simulink model "Final_V620140905h5b_fuben1"  (Simulink 7.9)
settings: Solver=FixedStepDiscrete  StartTime=0.0  StopTime=1  FixedStep=Auto  RelTol=1e-3
undefined symbols (not defined in the file or in its folder): Down, Up
libraries: tiiqmathlib x157, idelinklib_common x83, c2833xlib x37, simulink x12, c28xdmclib x12, c280xlib x7, simulink_extras x4, commutil2 x2, idelinklib_tgtpref x1, idelinklib_ticcs x1
(part 3 of 7)

== system Final_V620140905h5b_fuben1/Subsystem ==
  D2B : commutil2/Integer to Bit Converter  nbits=8  signedInputValues=Unsigned  bitOrder=LSB first  outDtype=uint16
  Demux : Demux  Outputs=8
  Memory Allocate : idelinklib_common/Memory Allocate  variableName=temp  alignThisVariable=off  memoryAlignmentBoundary=4  dataType=uint8  specifyQualifier=off  typeQualifier=volatile  dataDimension=1  specifyMemorySection=off  memorySection=mySEC1  bindMemorySection=on  sectionStartAddress=hex2dec('8000')  initializeMemory=off  initialValue=0
  Memory Copy2 : idelinklib_common/Memory Copy  Priority=3  copyFrom=Specified address  copyFromAddressSource=Specify via dialog  copyFromAddress=hex2dec('20000c')  copyFromSrcCode=myVariableSrc  dataTypeFrom=uint8  dataDimensionFrom=1  useOffsetFrom=off  offsetFromSrc=Specify via dialog  offsetFrom=0  strideFrom=1  copyTo=Output port  copyToAddressSource=Specify via dialog  copyToAddress=temp  copyToSrcCode=temp  dataTypeTo=uint8  useOffsetTo=off  offsetToSrc=Specify via dialog  offsetTo=0  strideTo=1  sampleTime=inf  useInitValue=off  initValueSrc=Specify constant value  initValue=bin2dec('00000000')  initValueSrcCode=myInitValueVariable  useAsMask=off  maskOperator=bitwise AND  useTermValue=off  termValue=bin2dec('00000000')  isRealtimeEnabled=off  emitCCBeforeWrite=off  CCBeforeWrite=/* Custom Code Before Write*/  emitCCAfterWrite=off  CCAfterWrite=/* Custom Code After Write*/  useDMACopy=off  enableBlockingMode=off
  J11-3&J11-4 : Outport
  J11-1&J11-2 : Outport  Port=2
  J12-3&J12-4 : Outport  Port=3
  J12-1&J12-2 : Outport  Port=4
  J13-3&J13-4 : Outport  Port=5
  J13-1&J13-2 : Outport  Port=6
  J14-3&J14-4 : Outport  Port=7
  J14-1&J14-2 : Outport  Port=8
  wires:
  Memory Copy2/1 -> D2B/1
  D2B/1 -> Demux/1
  Demux/1 -> J11-3&J11-4/1
  Demux/2 -> J11-1&J11-2/1
  Demux/3 -> J12-3&J12-4/1
  Demux/4 -> J12-1&J12-2/1
  Demux/5 -> J13-3&J13-4/1
  Demux/6 -> J13-1&J13-2/1
  Demux/7 -> J14-3&J14-4/1
  Demux/8 -> J14-1&J14-2/1

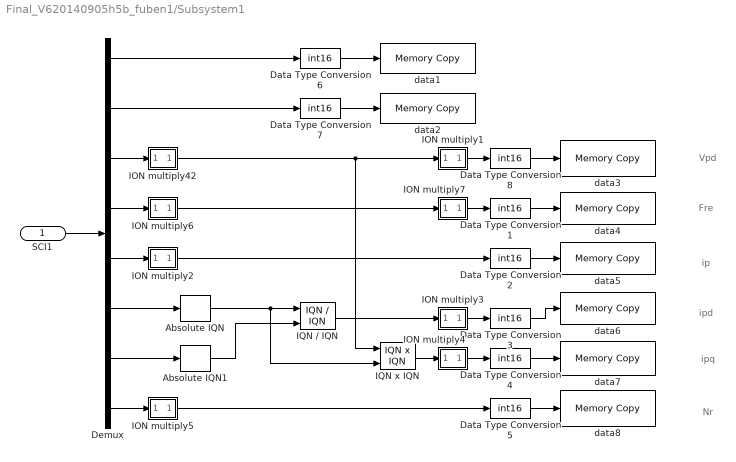
== system Final_V620140905h5b_fuben1/Subsystem1 ==
  note: Vpd
  note: Fre
  note: ip
  note: ipd
  note: ipq
  note: Nr
  SCI1 : Inport
  Absolute IQN : tiiqmathlib/Absolute IQN
  Absolute IQN1 : tiiqmathlib/Absolute IQN
  Data Type Conversion{1..8} (8 alike) : DataTypeConversion  OutDataTypeStr=int16
  Demux : Demux  Outputs=8
  ION multiply1 : Subsystem  mask{x=10}
      mask prompts: x "gain"
  ION multiply2 : Subsystem  mask{x=10}
      mask prompts: x "gain"
  ION multiply3 : Subsystem  mask{x=10}
      mask prompts: x "gain"
  ION multiply4 : Subsystem  mask{x=10}
      mask prompts: x "gain"
  ION multiply42 : Subsystem  mask{x=1.732/1.414}
      mask prompts: x "gain"
  ION multiply5 : Subsystem  mask{x=100}
      mask prompts: x "gain"
  ION multiply6 : Subsystem  mask{x=1.732/1.414}
      mask prompts: x "gain"
  ION multiply7 : Subsystem  mask{x=10}
      mask prompts: x "gain"
  IQN / IQN : tiiqmathlib/IQN // IQN
  IQN x IQN : tiiqmathlib/IQN x IQN  multiplyOption=Multiply
  data1 : idelinklib_common/Memory Copy  Priority=9  copyFrom=Input port  copyFromAddressSource=Specify via dialog  copyFromAddress=hex2dec('200004')  copyFromSrcCode=data  dataTypeFrom=int16  dataDimensionFrom=1  useOffsetFrom=off  offsetFromSrc=Specify via dialog  offsetFrom=0  strideFrom=1  copyTo=Specified source code symbol  copyToAddressSource=Specify via dialog  copyToAddress=temp  copyToSrcCode=data  dataTypeTo=int16  useOffsetTo=on  offsetToSrc=Specify via dialog  offsetTo=0  strideTo=1  sampleTime=inf  useInitValue=on  initValueSrc=Specify constant value  initValue=bin2dec('00000000')  initValueSrcCode=myInitValueVariable  useAsMask=off  maskOperator=bitwise AND  useTermValue=off  termValue=bin2dec('00000000')  isRealtimeEnabled=off  emitCCBeforeWrite=off  CCBeforeWrite=/* Custom Code Before Write*/  emitCCAfterWrite=off  CCAfterWrite=/* Custom Code After Write*/  useDMACopy=off  enableBlockingMode=off
  data2 : idelinklib_common/Memory Copy  Priority=9  copyFrom=Input port  copyFromAddressSource=Specify via dialog  copyFromAddress=hex2dec('200004')  copyFromSrcCode=data  dataTypeFrom=int16  dataDimensionFrom=1  useOffsetFrom=off  offsetFromSrc=Specify via dialog  offsetFrom=0  strideFrom=1  copyTo=Specified source code symbol  copyToAddressSource=Specify via dialog  copyToAddress=temp  copyToSrcCode=data  dataTypeTo=int16  useOffsetTo=on  offsetToSrc=Specify via dialog  offsetTo=1  strideTo=1  sampleTime=inf  useInitValue=on  initValueSrc=Specify constant value  initValue=bin2dec('00000000')  initValueSrcCode=myInitValueVariable  useAsMask=off  maskOperator=bitwise AND  useTermValue=off  termValue=bin2dec('00000000')  isRealtimeEnabled=off  emitCCBeforeWrite=off  CCBeforeWrite=/* Custom Code Before Write*/  emitCCAfterWrite=off  CCAfterWrite=/* Custom Code After Write*/  useDMACopy=off  enableBlockingMode=off
  data3 : idelinklib_common/Memory Copy  Priority=9  copyFrom=Input port  copyFromAddressSource=Specify via dialog  copyFromAddress=hex2dec('200004')  copyFromSrcCode=data  dataTypeFrom=int16  dataDimensionFrom=1  useOffsetFrom=off  offsetFromSrc=Specify via dialog  offsetFrom=0  strideFrom=1  copyTo=Specified source code symbol  copyToAddressSource=Specify via dialog  copyToAddress=temp  copyToSrcCode=data  dataTypeTo=int16  useOffsetTo=on  offsetToSrc=Specify via dialog  offsetTo=2  strideTo=1  sampleTime=inf  useInitValue=on  initValueSrc=Specify constant value  initValue=bin2dec('00000000')  initValueSrcCode=myInitValueVariable  useAsMask=off  maskOperator=bitwise AND  useTermValue=off  termValue=bin2dec('00000000')  isRealtimeEnabled=off  emitCCBeforeWrite=off  CCBeforeWrite=/* Custom Code Before Write*/  emitCCAfterWrite=off  CCAfterWrite=/* Custom Code After Write*/  useDMACopy=off  enableBlockingMode=off
  data4 : idelinklib_common/Memory Copy  Priority=9  copyFrom=Input port  copyFromAddressSource=Specify via dialog  copyFromAddress=hex2dec('200004')  copyFromSrcCode=data  dataTypeFrom=int16  dataDimensionFrom=1  useOffsetFrom=off  offsetFromSrc=Specify via dialog  offsetFrom=0  strideFrom=1  copyTo=Specified source code symbol  copyToAddressSource=Specify via dialog  copyToAddress=temp  copyToSrcCode=data  dataTypeTo=int16  useOffsetTo=on  offsetToSrc=Specify via dialog  offsetTo=3  strideTo=1  sampleTime=inf  useInitValue=on  initValueSrc=Specify constant value  initValue=bin2dec('00000000')  initValueSrcCode=myInitValueVariable  useAsMask=off  maskOperator=bitwise AND  useTermValue=off  termValue=bin2dec('00000000')  isRealtimeEnabled=off  emitCCBeforeWrite=off  CCBeforeWrite=/* Custom Code Before Write*/  emitCCAfterWrite=off  CCAfterWrite=/* Custom Code After Write*/  useDMACopy=off  enableBlockingMode=off
  data5 : idelinklib_common/Memory Copy  Priority=9  copyFrom=Input port  copyFromAddressSource=Specify via dialog  copyFromAddress=hex2dec('200004')  copyFromSrcCode=data  dataTypeFrom=int16  dataDimensionFrom=1  useOffsetFrom=off  offsetFromSrc=Specify via dialog  offsetFrom=0  strideFrom=1  copyTo=Specified source code symbol  copyToAddressSource=Specify via dialog  copyToAddress=temp  copyToSrcCode=data  dataTypeTo=int16  useOffsetTo=on  offsetToSrc=Specify via dialog  offsetTo=4  strideTo=1  sampleTime=inf  useInitValue=off  initValueSrc=Specify constant value  initValue=bin2dec('00000000')  initValueSrcCode=myInitValueVariable  useAsMask=off  maskOperator=bitwise AND  useTermValue=off  termValue=bin2dec('00000000')  isRealtimeEnabled=off  emitCCBeforeWrite=off  CCBeforeWrite=/* Custom Code Before Write*/  emitCCAfterWrite=off  CCAfterWrite=/* Custom Code After Write*/  useDMACopy=off  enableBlockingMode=off
  data6 : idelinklib_common/Memory Copy  Priority=9  copyFrom=Input port  copyFromAddressSource=Specify via dialog  copyFromAddress=hex2dec('200004')  copyFromSrcCode=data  dataTypeFrom=int16  dataDimensionFrom=1  useOffsetFrom=off  offsetFromSrc=Specify via dialog  offsetFrom=0  strideFrom=1  copyTo=Specified source code symbol  copyToAddressSource=Specify via dialog  copyToAddress=temp  copyToSrcCode=data  dataTypeTo=int16  useOffsetTo=on  offsetToSrc=Specify via dialog  offsetTo=5  strideTo=1  sampleTime=inf  useInitValue=on  initValueSrc=Specify constant value  initValue=bin2dec('00000000')  initValueSrcCode=myInitValueVariable  useAsMask=off  maskOperator=bitwise AND  useTermValue=off  termValue=bin2dec('00000000')  isRealtimeEnabled=off  emitCCBeforeWrite=off  CCBeforeWrite=/* Custom Code Before Write*/  emitCCAfterWrite=off  CCAfterWrite=/* Custom Code After Write*/  useDMACopy=off  enableBlockingMode=off
  data7 : idelinklib_common/Memory Copy  Priority=9  copyFrom=Input port  copyFromAddressSource=Specify via dialog  copyFromAddress=hex2dec('200004')  copyFromSrcCode=data  dataTypeFrom=int16  dataDimensionFrom=1  useOffsetFrom=off  offsetFromSrc=Specify via dialog  offsetFrom=0  strideFrom=1  copyTo=Specified source code symbol  copyToAddressSource=Specify via dialog  copyToAddress=temp  copyToSrcCode=data  dataTypeTo=int16  useOffsetTo=on  offsetToSrc=Specify via dialog  offsetTo=6  strideTo=1  sampleTime=inf  useInitValue=on  initValueSrc=Specify constant value  initValue=bin2dec('00000000')  initValueSrcCode=myInitValueVariable  useAsMask=off  maskOperator=bitwise AND  useTermValue=off  termValue=bin2dec('00000000')  isRealtimeEnabled=off  emitCCBeforeWrite=off  CCBeforeWrite=/* Custom Code Before Write*/  emitCCAfterWrite=off  CCAfterWrite=/* Custom Code After Write*/  useDMACopy=off  enableBlockingMode=off
  data8 : idelinklib_common/Memory Copy  Priority=9  copyFrom=Input port  copyFromAddressSource=Specify via dialog  copyFromAddress=hex2dec('200004')  copyFromSrcCode=data  dataTypeFrom=int16  dataDimensionFrom=1  useOffsetFrom=off  offsetFromSrc=Specify via dialog  offsetFrom=0  strideFrom=1  copyTo=Specified source code symbol  copyToAddressSource=Specify via dialog  copyToAddress=temp  copyToSrcCode=data  dataTypeTo=int16  useOffsetTo=on  offsetToSrc=Specify via dialog  offsetTo=7  strideTo=1  sampleTime=inf  useInitValue=on  initValueSrc=Specify constant value  initValue=bin2dec('00000000')  initValueSrcCode=myInitValueVariable  useAsMask=off  maskOperator=bitwise AND  useTermValue=off  termValue=bin2dec('00000000')  isRealtimeEnabled=off  emitCCBeforeWrite=off  CCBeforeWrite=/* Custom Code Before Write*/  emitCCAfterWrite=off  CCAfterWrite=/* Custom Code After Write*/  useDMACopy=off  enableBlockingMode=off
  wires:
  Data Type Conversion3/1 -> data6/1
  Data Type Conversion4/1 -> data7/1
  Data Type Conversion5/1 -> data8/1
  Data Type Conversion8/1 -> data3/1
  Data Type Conversion1/1 -> data4/1
  Data Type Conversion2/1 -> data5/1
  SCI1/1 -> Demux/1
  Demux/5 -> ION multiply2/1(x)
  Demux/8 -> ION multiply5/1(x)
  Demux/3 -> ION multiply42/1(x)
  Demux/1 -> Data Type Conversion6/1
  Demux/2 -> Data Type Conversion7/1
  ION multiply42/1(Kx) -> ION multiply1/1(x), IQN x IQN/1
  ION multiply1/1(Kx) -> Data Type Conversion8/1
  ION multiply2/1(Kx) -> Data Type Conversion2/1
  Demux/6 -> Absolute IQN/1
  Demux/7 -> Absolute IQN1/1
  Absolute IQN/1 -> IQN / IQN/1, IQN x IQN/2
  Absolute IQN1/1 -> IQN / IQN/2
  IQN / IQN/1 -> ION multiply3/1(x)
  ION multiply3/1(Kx) -> Data Type Conversion3/1
  ION multiply4/1(Kx) -> Data Type Conversion4/1
  IQN x IQN/1 -> ION multiply4/1(x)
  ION multiply5/1(Kx) -> Data Type Conversion5/1
  Demux/4 -> ION multiply6/1(x)
  ION multiply7/1(Kx) -> Data Type Conversion1/1
  Data Type Conversion6/1 -> data1/1
  Data Type Conversion7/1 -> data2/1
  ION multiply6/1(Kx) -> ION multiply7/1(x)

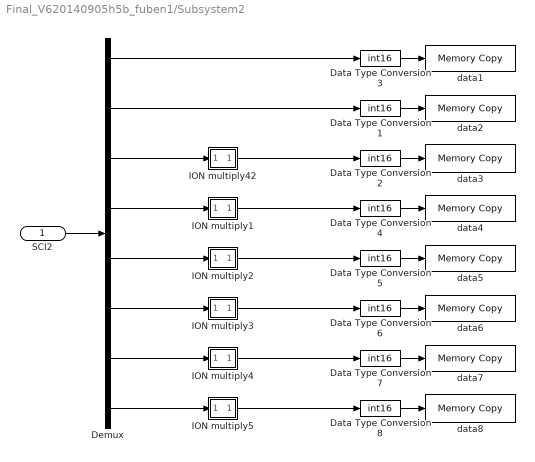
== system Final_V620140905h5b_fuben1/Subsystem2 ==
  SCI2 : Inport
  Data Type Conversion{1..8} (8 alike) : DataTypeConversion  OutDataTypeStr=int16
  Demux : Demux  Outputs=8
  ION multiply1 : Subsystem  mask{x=100}
      mask prompts: x "gain"
  ION multiply2 : Subsystem  mask{x=100}
      mask prompts: x "gain"
  ION multiply3 : Subsystem  mask{x=10}
      mask prompts: x "gain"
  ION multiply4 : Subsystem  mask{x=10}
      mask prompts: x "gain"
  ION multiply42 : Subsystem  mask{x=100}
      mask prompts: x "gain"
  ION multiply5 : Subsystem  mask{x=10}
      mask prompts: x "gain"
  data1 : idelinklib_common/Memory Copy  Priority=9  copyFrom=Input port  copyFromAddressSource=Specify via dialog  copyFromAddress=hex2dec('200004')  copyFromSrcCode=data  dataTypeFrom=int16  dataDimensionFrom=1  useOffsetFrom=off  offsetFromSrc=Specify via dialog  offsetFrom=0  strideFrom=1  copyTo=Specified source code symbol  copyToAddressSource=Specify via dialog  copyToAddress=temp  copyToSrcCode=data1  dataTypeTo=int16  useOffsetTo=on  offsetToSrc=Specify via dialog  offsetTo=0  strideTo=1  sampleTime=inf  useInitValue=on  initValueSrc=Specify constant value  initValue=bin2dec('00000000')  initValueSrcCode=myInitValueVariable  useAsMask=off  maskOperator=bitwise AND  useTermValue=off  termValue=bin2dec('00000000')  isRealtimeEnabled=off  emitCCBeforeWrite=off  CCBeforeWrite=/* Custom Code Before Write*/  emitCCAfterWrite=off  CCAfterWrite=/* Custom Code After Write*/  useDMACopy=off  enableBlockingMode=off
  data2 : idelinklib_common/Memory Copy  Priority=9  copyFrom=Input port  copyFromAddressSource=Specify via dialog  copyFromAddress=hex2dec('200004')  copyFromSrcCode=data  dataTypeFrom=int16  dataDimensionFrom=1  useOffsetFrom=off  offsetFromSrc=Specify via dialog  offsetFrom=0  strideFrom=1  copyTo=Specified source code symbol  copyToAddressSource=Specify via dialog  copyToAddress=temp  copyToSrcCode=data1  dataTypeTo=int16  useOffsetTo=on  offsetToSrc=Specify via dialog  offsetTo=1  strideTo=1  sampleTime=inf  useInitValue=on  initValueSrc=Specify constant value  initValue=bin2dec('00000000')  initValueSrcCode=myInitValueVariable  useAsMask=off  maskOperator=bitwise AND  useTermValue=off  termValue=bin2dec('00000000')  isRealtimeEnabled=off  emitCCBeforeWrite=off  CCBeforeWrite=/* Custom Code Before Write*/  emitCCAfterWrite=off  CCAfterWrite=/* Custom Code After Write*/  useDMACopy=off  enableBlockingMode=off
  data3 : idelinklib_common/Memory Copy  Priority=9  copyFrom=Input port  copyFromAddressSource=Specify via dialog  copyFromAddress=hex2dec('200004')  copyFromSrcCode=data  dataTypeFrom=int16  dataDimensionFrom=1  useOffsetFrom=off  offsetFromSrc=Specify via dialog  offsetFrom=0  strideFrom=1  copyTo=Specified source code symbol  copyToAddressSource=Specify via dialog  copyToAddress=temp  copyToSrcCode=data1  dataTypeTo=int16  useOffsetTo=on  offsetToSrc=Specify via dialog  offsetTo=2  strideTo=1  sampleTime=inf  useInitValue=on  initValueSrc=Specify constant value  initValue=bin2dec('00000000')  initValueSrcCode=myInitValueVariable  useAsMask=off  maskOperator=bitwise AND  useTermValue=off  termValue=bin2dec('00000000')  isRealtimeEnabled=off  emitCCBeforeWrite=off  CCBeforeWrite=/* Custom Code Before Write*/  emitCCAfterWrite=off  CCAfterWrite=/* Custom Code After Write*/  useDMACopy=off  enableBlockingMode=off
  data4 : idelinklib_common/Memory Copy  Priority=9  copyFrom=Input port  copyFromAddressSource=Specify via dialog  copyFromAddress=hex2dec('200004')  copyFromSrcCode=data  dataTypeFrom=int16  dataDimensionFrom=1  useOffsetFrom=off  offsetFromSrc=Specify via dialog  offsetFrom=0  strideFrom=1  copyTo=Specified source code symbol  copyToAddressSource=Specify via dialog  copyToAddress=temp  copyToSrcCode=data1  dataTypeTo=int16  useOffsetTo=on  offsetToSrc=Specify via dialog  offsetTo=3  strideTo=1  sampleTime=inf  useInitValue=on  initValueSrc=Specify constant value  initValue=bin2dec('00000000')  initValueSrcCode=myInitValueVariable  useAsMask=off  maskOperator=bitwise AND  useTermValue=off  termValue=bin2dec('00000000')  isRealtimeEnabled=off  emitCCBeforeWrite=off  CCBeforeWrite=/* Custom Code Before Write*/  emitCCAfterWrite=off  CCAfterWrite=/* Custom Code After Write*/  useDMACopy=off  enableBlockingMode=off
  data5 : idelinklib_common/Memory Copy  Priority=9  copyFrom=Input port  copyFromAddressSource=Specify via dialog  copyFromAddress=hex2dec('200004')  copyFromSrcCode=data  dataTypeFrom=int16  dataDimensionFrom=1  useOffsetFrom=off  offsetFromSrc=Specify via dialog  offsetFrom=0  strideFrom=1  copyTo=Specified source code symbol  copyToAddressSource=Specify via dialog  copyToAddress=temp  copyToSrcCode=data1  dataTypeTo=int16  useOffsetTo=on  offsetToSrc=Specify via dialog  offsetTo=4  strideTo=1  sampleTime=inf  useInitValue=off  initValueSrc=Specify constant value  initValue=bin2dec('00000000')  initValueSrcCode=myInitValueVariable  useAsMask=off  maskOperator=bitwise AND  useTermValue=off  termValue=bin2dec('00000000')  isRealtimeEnabled=off  emitCCBeforeWrite=off  CCBeforeWrite=/* Custom Code Before Write*/  emitCCAfterWrite=off  CCAfterWrite=/* Custom Code After Write*/  useDMACopy=off  enableBlockingMode=off
  data6 : idelinklib_common/Memory Copy  Priority=9  copyFrom=Input port  copyFromAddressSource=Specify via dialog  copyFromAddress=hex2dec('200004')  copyFromSrcCode=data  dataTypeFrom=int16  dataDimensionFrom=1  useOffsetFrom=off  offsetFromSrc=Specify via dialog  offsetFrom=0  strideFrom=1  copyTo=Specified source code symbol  copyToAddressSource=Specify via dialog  copyToAddress=temp  copyToSrcCode=data1  dataTypeTo=int16  useOffsetTo=on  offsetToSrc=Specify via dialog  offsetTo=5  strideTo=1  sampleTime=inf  useInitValue=on  initValueSrc=Specify constant value  initValue=bin2dec('00000000')  initValueSrcCode=myInitValueVariable  useAsMask=off  maskOperator=bitwise AND  useTermValue=off  termValue=bin2dec('00000000')  isRealtimeEnabled=off  emitCCBeforeWrite=off  CCBeforeWrite=/* Custom Code Before Write*/  emitCCAfterWrite=off  CCAfterWrite=/* Custom Code After Write*/  useDMACopy=off  enableBlockingMode=off
  data7 : idelinklib_common/Memory Copy  Priority=9  copyFrom=Input port  copyFromAddressSource=Specify via dialog  copyFromAddress=hex2dec('200004')  copyFromSrcCode=data  dataTypeFrom=int16  dataDimensionFrom=1  useOffsetFrom=off  offsetFromSrc=Specify via dialog  offsetFrom=0  strideFrom=1  copyTo=Specified source code symbol  copyToAddressSource=Specify via dialog  copyToAddress=temp  copyToSrcCode=data1  dataTypeTo=int16  useOffsetTo=on  offsetToSrc=Specify via dialog  offsetTo=6  strideTo=1  sampleTime=inf  useInitValue=on  initValueSrc=Specify constant value  initValue=bin2dec('00000000')  initValueSrcCode=myInitValueVariable  useAsMask=off  maskOperator=bitwise AND  useTermValue=off  termValue=bin2dec('00000000')  isRealtimeEnabled=off  emitCCBeforeWrite=off  CCBeforeWrite=/* Custom Code Before Write*/  emitCCAfterWrite=off  CCAfterWrite=/* Custom Code After Write*/  useDMACopy=off  enableBlockingMode=off
  data8 : idelinklib_common/Memory Copy  Priority=9  copyFrom=Input port  copyFromAddressSource=Specify via dialog  copyFromAddress=hex2dec('200004')  copyFromSrcCode=data  dataTypeFrom=int16  dataDimensionFrom=1  useOffsetFrom=off  offsetFromSrc=Specify via dialog  offsetFrom=0  strideFrom=1  copyTo=Specified source code symbol  copyToAddressSource=Specify via dialog  copyToAddress=temp  copyToSrcCode=data1  dataTypeTo=int16  useOffsetTo=on  offsetToSrc=Specify via dialog  offsetTo=7  strideTo=1  sampleTime=inf  useInitValue=on  initValueSrc=Specify constant value  initValue=bin2dec('00000000')  initValueSrcCode=myInitValueVariable  useAsMask=off  maskOperator=bitwise AND  useTermValue=off  termValue=bin2dec('00000000')  isRealtimeEnabled=off  emitCCBeforeWrite=off  CCBeforeWrite=/* Custom Code Before Write*/  emitCCAfterWrite=off  CCAfterWrite=/* Custom Code After Write*/  useDMACopy=off  enableBlockingMode=off
  wires:
  SCI2/1 -> Demux/1
  Demux/4 -> ION multiply1/1(x)
  Demux/5 -> ION multiply2/1(x)
  Demux/7 -> ION multiply4/1(x)
  Data Type Conversion3/1 -> data1/1
  Data Type Conversion1/1 -> data2/1
  Data Type Conversion2/1 -> data3/1
  Data Type Conversion4/1 -> data4/1
  Data Type Conversion5/1 -> data5/1
  Data Type Conversion6/1 -> data6/1
  Data Type Conversion7/1 -> data7/1
  Data Type Conversion8/1 -> data8/1
  Demux/8 -> ION multiply5/1(x)
  Demux/1 -> Data Type Conversion3/1
  Demux/2 -> Data Type Conversion1/1
  Demux/3 -> ION multiply42/1(x)
  Demux/6 -> ION multiply3/1(x)
  ION multiply5/1(Kx) -> Data Type Conversion8/1
  ION multiply42/1(Kx) -> Data Type Conversion2/1
  ION multiply1/1(Kx) -> Data Type Conversion4/1
  ION multiply2/1(Kx) -> Data Type Conversion5/1
  ION multiply3/1(Kx) -> Data Type Conversion6/1
  ION multiply4/1(Kx) -> Data Type Conversion7/1

== system Final_V620140905h5b_fuben1/Subsystem3 ==
  note: ipd
  note: Md
  note: icd
  note: ipq
  note: Mq
  note: state
  SCI3 : Inport
  Data Type Conversion{1..8} (8 alike) : DataTypeConversion  OutDataTypeStr=int16
  Demux : Demux  Outputs=8
  ION multiply1 : Subsystem  mask{x=10}
      mask prompts: x "gain"
  ION multiply2 : Subsystem  mask{x=10}
      mask prompts: x "gain"
  ION multiply3 : Subsystem  mask{x=10}
      mask prompts: x "gain"
  ION multiply4 : Subsystem  mask{x=10}
      mask prompts: x "gain"
  ION multiply5 : Subsystem  mask{x=10}
      mask prompts: x "gain"
  data1 : idelinklib_common/Memory Copy  Priority=9  copyFrom=Input port  copyFromAddressSource=Specify via dialog  copyFromAddress=hex2dec('200004')  copyFromSrcCode=data  dataTypeFrom=int16  dataDimensionFrom=1  useOffsetFrom=off  offsetFromSrc=Specify via dialog  offsetFrom=0  strideFrom=1  copyTo=Specified source code symbol  copyToAddressSource=Specify via dialog  copyToAddress=temp  copyToSrcCode=data2  dataTypeTo=int16  useOffsetTo=on  offsetToSrc=Specify via dialog  offsetTo=0  strideTo=1  sampleTime=inf  useInitValue=on  initValueSrc=Specify constant value  initValue=bin2dec('00000000')  initValueSrcCode=myInitValueVariable  useAsMask=off  maskOperator=bitwise AND  useTermValue=off  termValue=bin2dec('00000000')  isRealtimeEnabled=off  emitCCBeforeWrite=off  CCBeforeWrite=/* Custom Code Before Write*/  emitCCAfterWrite=off  CCAfterWrite=/* Custom Code After Write*/  useDMACopy=off  enableBlockingMode=off
  data2 : idelinklib_common/Memory Copy  Priority=9  copyFrom=Input port  copyFromAddressSource=Specify via dialog  copyFromAddress=hex2dec('200004')  copyFromSrcCode=data  dataTypeFrom=int16  dataDimensionFrom=1  useOffsetFrom=off  offsetFromSrc=Specify via dialog  offsetFrom=0  strideFrom=1  copyTo=Specified source code symbol  copyToAddressSource=Specify via dialog  copyToAddress=temp  copyToSrcCode=data2  dataTypeTo=int16  useOffsetTo=on  offsetToSrc=Specify via dialog  offsetTo=1  strideTo=1  sampleTime=inf  useInitValue=on  initValueSrc=Specify constant value  initValue=bin2dec('00000000')  initValueSrcCode=myInitValueVariable  useAsMask=off  maskOperator=bitwise AND  useTermValue=off  termValue=bin2dec('00000000')  isRealtimeEnabled=off  emitCCBeforeWrite=off  CCBeforeWrite=/* Custom Code Before Write*/  emitCCAfterWrite=off  CCAfterWrite=/* Custom Code After Write*/  useDMACopy=off  enableBlockingMode=off
  data3 : idelinklib_common/Memory Copy  Priority=9  copyFrom=Input port  copyFromAddressSource=Specify via dialog  copyFromAddress=hex2dec('200004')  copyFromSrcCode=data  dataTypeFrom=int16  dataDimensionFrom=1  useOffsetFrom=off  offsetFromSrc=Specify via dialog  offsetFrom=0  strideFrom=1  copyTo=Specified source code symbol  copyToAddressSource=Specify via dialog  copyToAddress=temp  copyToSrcCode=data2  dataTypeTo=int16  useOffsetTo=on  offsetToSrc=Specify via dialog  offsetTo=2  strideTo=1  sampleTime=inf  useInitValue=on  initValueSrc=Specify constant value  initValue=bin2dec('00000000')  initValueSrcCode=myInitValueVariable  useAsMask=off  maskOperator=bitwise AND  useTermValue=off  termValue=bin2dec('00000000')  isRealtimeEnabled=off  emitCCBeforeWrite=off  CCBeforeWrite=/* Custom Code Before Write*/  emitCCAfterWrite=off  CCAfterWrite=/* Custom Code After Write*/  useDMACopy=off  enableBlockingMode=off
  data4 : idelinklib_common/Memory Copy  Priority=9  copyFrom=Input port  copyFromAddressSource=Specify via dialog  copyFromAddress=hex2dec('200004')  copyFromSrcCode=data  dataTypeFrom=int16  dataDimensionFrom=1  useOffsetFrom=off  offsetFromSrc=Specify via dialog  offsetFrom=0  strideFrom=1  copyTo=Specified source code symbol  copyToAddressSource=Specify via dialog  copyToAddress=temp  copyToSrcCode=data2  dataTypeTo=int16  useOffsetTo=on  offsetToSrc=Specify via dialog  offsetTo=3  strideTo=1  sampleTime=inf  useInitValue=on  initValueSrc=Specify constant value  initValue=bin2dec('00000000')  initValueSrcCode=myInitValueVariable  useAsMask=off  maskOperator=bitwise AND  useTermValue=off  termValue=bin2dec('00000000')  isRealtimeEnabled=off  emitCCBeforeWrite=off  CCBeforeWrite=/* Custom Code Before Write*/  emitCCAfterWrite=off  CCAfterWrite=/* Custom Code After Write*/  useDMACopy=off  enableBlockingMode=off
  data5 : idelinklib_common/Memory Copy  Priority=9  copyFrom=Input port  copyFromAddressSource=Specify via dialog  copyFromAddress=hex2dec('200004')  copyFromSrcCode=data  dataTypeFrom=int16  dataDimensionFrom=1  useOffsetFrom=off  offsetFromSrc=Specify via dialog  offsetFrom=0  strideFrom=1  copyTo=Specified source code symbol  copyToAddressSource=Specify via dialog  copyToAddress=temp  copyToSrcCode=data2  dataTypeTo=int16  useOffsetTo=on  offsetToSrc=Specify via dialog  offsetTo=4  strideTo=1  sampleTime=inf  useInitValue=off  initValueSrc=Specify constant value  initValue=bin2dec('00000000')  initValueSrcCode=myInitValueVariable  useAsMask=off  maskOperator=bitwise AND  useTermValue=off  termValue=bin2dec('00000000')  isRealtimeEnabled=off  emitCCBeforeWrite=off  CCBeforeWrite=/* Custom Code Before Write*/  emitCCAfterWrite=off  CCAfterWrite=/* Custom Code After Write*/  useDMACopy=off  enableBlockingMode=off
  data6 : idelinklib_common/Memory Copy  Priority=9  copyFrom=Input port  copyFromAddressSource=Specify via dialog  copyFromAddress=hex2dec('200004')  copyFromSrcCode=data  dataTypeFrom=int16  dataDimensionFrom=1  useOffsetFrom=off  offsetFromSrc=Specify via dialog  offsetFrom=0  strideFrom=1  copyTo=Specified source code symbol  copyToAddressSource=Specify via dialog  copyToAddress=temp  copyToSrcCode=data2  dataTypeTo=int16  useOffsetTo=on  offsetToSrc=Specify via dialog  offsetTo=5  strideTo=1  sampleTime=inf  useInitValue=on  initValueSrc=Specify constant value  initValue=bin2dec('00000000')  initValueSrcCode=myInitValueVariable  useAsMask=off  maskOperator=bitwise AND  useTermValue=off  termValue=bin2dec('00000000')  isRealtimeEnabled=off  emitCCBeforeWrite=off  CCBeforeWrite=/* Custom Code Before Write*/  emitCCAfterWrite=off  CCAfterWrite=/* Custom Code After Write*/  useDMACopy=off  enableBlockingMode=off
  data7 : idelinklib_common/Memory Copy  Priority=9  copyFrom=Input port  copyFromAddressSource=Specify via dialog  copyFromAddress=hex2dec('200004')  copyFromSrcCode=data  dataTypeFrom=int16  dataDimensionFrom=1  useOffsetFrom=off  offsetFromSrc=Specify via dialog  offsetFrom=0  strideFrom=1  copyTo=Specified source code symbol  copyToAddressSource=Specify via dialog  copyToAddress=temp  copyToSrcCode=data2  dataTypeTo=int16  useOffsetTo=on  offsetToSrc=Specify via dialog  offsetTo=6  strideTo=1  sampleTime=inf  useInitValue=on  initValueSrc=Specify constant value  initValue=bin2dec('00000000')  initValueSrcCode=myInitValueVariable  useAsMask=off  maskOperator=bitwise AND  useTermValue=off  termValue=bin2dec('00000000')  isRealtimeEnabled=off  emitCCBeforeWrite=off  CCBeforeWrite=/* Custom Code Before Write*/  emitCCAfterWrite=off  CCAfterWrite=/* Custom Code After Write*/  useDMACopy=off  enableBlockingMode=off
  data8 : idelinklib_common/Memory Copy  Priority=9  copyFrom=Input port  copyFromAddressSource=Specify via dialog  copyFromAddress=hex2dec('200004')  copyFromSrcCode=data  dataTypeFrom=int16  dataDimensionFrom=1  useOffsetFrom=off  offsetFromSrc=Specify via dialog  offsetFrom=0  strideFrom=1  copyTo=Specified source code symbol  copyToAddressSource=Specify via dialog  copyToAddress=temp  copyToSrcCode=data2  dataTypeTo=int16  useOffsetTo=on  offsetToSrc=Specify via dialog  offsetTo=7  strideTo=1  sampleTime=inf  useInitValue=on  initValueSrc=Specify constant value  initValue=bin2dec('00000000')  initValueSrcCode=myInitValueVariable  useAsMask=off  maskOperator=bitwise AND  useTermValue=off  termValue=bin2dec('00000000')  isRealtimeEnabled=off  emitCCBeforeWrite=off  CCBeforeWrite=/* Custom Code Before Write*/  emitCCAfterWrite=off  CCAfterWrite=/* Custom Code After Write*/  useDMACopy=off  enableBlockingMode=off
  wires:
  Demux/1 -> Data Type Conversion3/1
  Demux/2 -> Data Type Conversion1/1
  SCI3/1 -> Demux/1
  Data Type Conversion3/1 -> data1/1
  Data Type Conversion1/1 -> data2/1
  Data Type Conversion2/1 -> data3/1
  Data Type Conversion4/1 -> data4/1
  Data Type Conversion5/1 -> data5/1
  Data Type Conversion6/1 -> data6/1
  Data Type Conversion7/1 -> data7/1
  Data Type Conversion8/1 -> data8/1
  Demux/5 -> ION multiply3/1(x)
  Demux/8 -> Data Type Conversion8/1
  Demux/3 -> ION multiply1/1(x)
  Demux/7 -> ION multiply5/1(x)
  ION multiply1/1(Kx) -> Data Type Conversion2/1
  Demux/4 -> ION multiply2/1(x)
  Demux/6 -> ION multiply4/1(x)
  ION multiply5/1(Kx) -> Data Type Conversion7/1
  ION multiply2/1(Kx) -> Data Type Conversion4/1
  ION multiply3/1(Kx) -> Data Type Conversion5/1
  ION multiply4/1(Kx) -> Data Type Conversion6/1

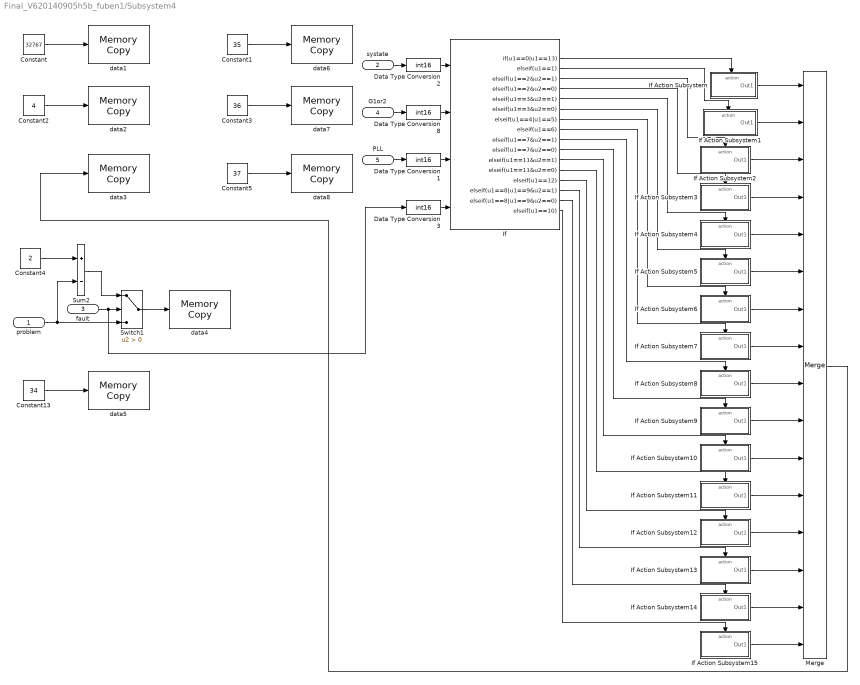
== system Final_V620140905h5b_fuben1/Subsystem4 ==
  problem : Inport
  systate : Inport  Port=2
  fault : Inport  Port=3
  G1or2 : Inport  Port=4
  PLL : Inport  Port=5
  Constant : Constant  Value=32767  OutDataTypeStr=int16
  Constant1 : Constant  Value=35  OutDataTypeStr=int16
  Constant13 : Constant  Value=34  OutDataTypeStr=int16
  Constant2 : Constant  Value=4  OutDataTypeStr=int16
  Constant3 : Constant  Value=36  OutDataTypeStr=int16
  Constant4 : Constant  Value=2  OutDataTypeStr=int16
  Constant5 : Constant  Value=37  OutDataTypeStr=int16
  Data Type Conversion{1..3,8} (4 alike) : DataTypeConversion  OutDataTypeStr=int16
  If : If  NumInputs=4  IfExpression=u1==0|u1==13  ElseIfExpressions=u1==1,u1==2&u2==1,u1==2&u2==0,u1==3&u2==1,u1==3&u2==0,u1==4|u1==5,u1==6,u1==7&u2==1,u1==7&u2==0,u1==11&u2==1,u1==11&u2==0,u1==12,u1==8|u1==9&u2==1,u1==8|u1==9&u2==0,u1==10  ShowElse=off
  If Action Subsystem : Subsystem  TreatAsAtomicUnit=on
  If Action Subsystem1 : Subsystem  TreatAsAtomicUnit=on
  If Action Subsystem10 : Subsystem  TreatAsAtomicUnit=on
  If Action Subsystem11 : Subsystem  TreatAsAtomicUnit=on
  If Action Subsystem12 : Subsystem  TreatAsAtomicUnit=on
  If Action Subsystem13 : Subsystem  TreatAsAtomicUnit=on
  If Action Subsystem14 : Subsystem  TreatAsAtomicUnit=on
  If Action Subsystem15 : Subsystem  TreatAsAtomicUnit=on
  If Action Subsystem2 : Subsystem  TreatAsAtomicUnit=on
  If Action Subsystem3 : Subsystem  TreatAsAtomicUnit=on
  If Action Subsystem4 : Subsystem  TreatAsAtomicUnit=on
  If Action Subsystem5 : Subsystem  TreatAsAtomicUnit=on
  If Action Subsystem6 : Subsystem  TreatAsAtomicUnit=on
  If Action Subsystem7 : Subsystem  TreatAsAtomicUnit=on
  If Action Subsystem8 : Subsystem  TreatAsAtomicUnit=on
  If Action Subsystem9 : Subsystem  TreatAsAtomicUnit=on
  Merge : Merge  Inputs=16
  Sum2 : Sum  Inputs=+-
  Switch1 : Switch  Criteria=u2 > Threshold  SaturateOnIntegerOverflow=on  InputSameDT=on
  data1 : idelinklib_common/Memory Copy  Priority=9  copyFrom=Input port  copyFromAddressSource=Specify via dialog  copyFromAddress=hex2dec('200004')  copyFromSrcCode=data  dataTypeFrom=int16  dataDimensionFrom=1  useOffsetFrom=off  offsetFromSrc=Specify via dialog  offsetFrom=0  strideFrom=1  copyTo=Specified source code symbol  copyToAddressSource=Specify via dialog  copyToAddress=temp  copyToSrcCode=data3  dataTypeTo=int16  useOffsetTo=on  offsetToSrc=Specify via dialog  offsetTo=0  strideTo=1  sampleTime=inf  useInitValue=on  initValueSrc=Specify constant value  initValue=bin2dec('00000000')  initValueSrcCode=myInitValueVariable  useAsMask=off  maskOperator=bitwise AND  useTermValue=off  termValue=bin2dec('00000000')  isRealtimeEnabled=off  emitCCBeforeWrite=off  CCBeforeWrite=/* Custom Code Before Write*/  emitCCAfterWrite=off  CCAfterWrite=/* Custom Code After Write*/  useDMACopy=off  enableBlockingMode=off
  data2 : idelinklib_common/Memory Copy  Priority=9  copyFrom=Input port  copyFromAddressSource=Specify via dialog  copyFromAddress=hex2dec('200004')  copyFromSrcCode=data  dataTypeFrom=int16  dataDimensionFrom=1  useOffsetFrom=off  offsetFromSrc=Specify via dialog  offsetFrom=0  strideFrom=1  copyTo=Specified source code symbol  copyToAddressSource=Specify via dialog  copyToAddress=temp  copyToSrcCode=data3  dataTypeTo=int16  useOffsetTo=on  offsetToSrc=Specify via dialog  offsetTo=1  strideTo=1  sampleTime=inf  useInitValue=on  initValueSrc=Specify constant value  initValue=bin2dec('00000000')  initValueSrcCode=myInitValueVariable  useAsMask=off  maskOperator=bitwise AND  useTermValue=off  termValue=bin2dec('00000000')  isRealtimeEnabled=off  emitCCBeforeWrite=off  CCBeforeWrite=/* Custom Code Before Write*/  emitCCAfterWrite=off  CCAfterWrite=/* Custom Code After Write*/  useDMACopy=off  enableBlockingMode=off
  data3 : idelinklib_common/Memory Copy  Priority=9  copyFrom=Input port  copyFromAddressSource=Specify via dialog  copyFromAddress=hex2dec('200004')  copyFromSrcCode=data  dataTypeFrom=int16  dataDimensionFrom=1  useOffsetFrom=off  offsetFromSrc=Specify via dialog  offsetFrom=0  strideFrom=1  copyTo=Specified source code symbol  copyToAddressSource=Specify via dialog  copyToAddress=temp  copyToSrcCode=data3  dataTypeTo=int16  useOffsetTo=on  offsetToSrc=Specify via dialog  offsetTo=2  strideTo=1  sampleTime=inf  useInitValue=on  initValueSrc=Specify constant value  initValue=bin2dec('00000000')  initValueSrcCode=myInitValueVariable  useAsMask=off  maskOperator=bitwise AND  useTermValue=off  termValue=bin2dec('00000000')  isRealtimeEnabled=off  emitCCBeforeWrite=off  CCBeforeWrite=/* Custom Code Before Write*/  emitCCAfterWrite=off  CCAfterWrite=/* Custom Code After Write*/  useDMACopy=off  enableBlockingMode=off
  data4 : idelinklib_common/Memory Copy  Priority=9  copyFrom=Input port  copyFromAddressSource=Specify via dialog  copyFromAddress=hex2dec('200004')  copyFromSrcCode=data  dataTypeFrom=int16  dataDimensionFrom=1  useOffsetFrom=off  offsetFromSrc=Specify via dialog  offsetFrom=0  strideFrom=1  copyTo=Specified source code symbol  copyToAddressSource=Specify via dialog  copyToAddress=temp  copyToSrcCode=data3  dataTypeTo=int16  useOffsetTo=on  offsetToSrc=Specify via dialog  offsetTo=3  strideTo=1  sampleTime=inf  useInitValue=on  initValueSrc=Specify constant value  initValue=bin2dec('00000000')  initValueSrcCode=myInitValueVariable  useAsMask=off  maskOperator=bitwise AND  useTermValue=off  termValue=bin2dec('00000000')  isRealtimeEnabled=off  emitCCBeforeWrite=off  CCBeforeWrite=/* Custom Code Before Write*/  emitCCAfterWrite=off  CCAfterWrite=/* Custom Code After Write*/  useDMACopy=off  enableBlockingMode=off
  data5 : idelinklib_common/Memory Copy  Priority=9  copyFrom=Input port  copyFromAddressSource=Specify via dialog  copyFromAddress=hex2dec('200004')  copyFromSrcCode=data  dataTypeFrom=int16  dataDimensionFrom=1  useOffsetFrom=off  offsetFromSrc=Specify via dialog  offsetFrom=0  strideFrom=1  copyTo=Specified source code symbol  copyToAddressSource=Specify via dialog  copyToAddress=temp  copyToSrcCode=data3  dataTypeTo=int16  useOffsetTo=on  offsetToSrc=Specify via dialog  offsetTo=4  strideTo=1  sampleTime=inf  useInitValue=off  initValueSrc=Specify constant value  initValue=bin2dec('00000000')  initValueSrcCode=myInitValueVariable  useAsMask=off  maskOperator=bitwise AND  useTermValue=off  termValue=bin2dec('00000000')  isRealtimeEnabled=off  emitCCBeforeWrite=off  CCBeforeWrite=/* Custom Code Before Write*/  emitCCAfterWrite=off  CCAfterWrite=/* Custom Code After Write*/  useDMACopy=off  enableBlockingMode=off
  data6 : idelinklib_common/Memory Copy  Priority=9  copyFrom=Input port  copyFromAddressSource=Specify via dialog  copyFromAddress=hex2dec('200004')  copyFromSrcCode=data  dataTypeFrom=int16  dataDimensionFrom=1  useOffsetFrom=off  offsetFromSrc=Specify via dialog  offsetFrom=0  strideFrom=1  copyTo=Specified source code symbol  copyToAddressSource=Specify via dialog  copyToAddress=temp  copyToSrcCode=data3  dataTypeTo=int16  useOffsetTo=on  offsetToSrc=Specify via dialog  offsetTo=5  strideTo=1  sampleTime=inf  useInitValue=on  initValueSrc=Specify constant value  initValue=bin2dec('00000000')  initValueSrcCode=myInitValueVariable  useAsMask=off  maskOperator=bitwise AND  useTermValue=off  termValue=bin2dec('00000000')  isRealtimeEnabled=off  emitCCBeforeWrite=off  CCBeforeWrite=/* Custom Code Before Write*/  emitCCAfterWrite=off  CCAfterWrite=/* Custom Code After Write*/  useDMACopy=off  enableBlockingMode=off
  data7 : idelinklib_common/Memory Copy  Priority=9  copyFrom=Input port  copyFromAddressSource=Specify via dialog  copyFromAddress=hex2dec('200004')  copyFromSrcCode=data  dataTypeFrom=int16  dataDimensionFrom=1  useOffsetFrom=off  offsetFromSrc=Specify via dialog  offsetFrom=0  strideFrom=1  copyTo=Specified source code symbol  copyToAddressSource=Specify via dialog  copyToAddress=temp  copyToSrcCode=data3  dataTypeTo=int16  useOffsetTo=on  offsetToSrc=Specify via dialog  offsetTo=6  strideTo=1  sampleTime=inf  useInitValue=on  initValueSrc=Specify constant value  initValue=bin2dec('00000000')  initValueSrcCode=myInitValueVariable  useAsMask=off  maskOperator=bitwise AND  useTermValue=off  termValue=bin2dec('00000000')  isRealtimeEnabled=off  emitCCBeforeWrite=off  CCBeforeWrite=/* Custom Code Before Write*/  emitCCAfterWrite=off  CCAfterWrite=/* Custom Code After Write*/  useDMACopy=off  enableBlockingMode=off
  data8 : idelinklib_common/Memory Copy  Priority=9  copyFrom=Input port  copyFromAddressSource=Specify via dialog  copyFromAddress=hex2dec('200004')  copyFromSrcCode=data  dataTypeFrom=int16  dataDimensionFrom=1  useOffsetFrom=off  offsetFromSrc=Specify via dialog  offsetFrom=0  strideFrom=1  copyTo=Specified source code symbol  copyToAddressSource=Specify via dialog  copyToAddress=temp  copyToSrcCode=data3  dataTypeTo=int16  useOffsetTo=on  offsetToSrc=Specify via dialog  offsetTo=7  strideTo=1  sampleTime=inf  useInitValue=on  initValueSrc=Specify constant value  initValue=bin2dec('00000000')  initValueSrcCode=myInitValueVariable  useAsMask=off  maskOperator=bitwise AND  useTermValue=off  termValue=bin2dec('00000000')  isRealtimeEnabled=off  emitCCBeforeWrite=off  CCBeforeWrite=/* Custom Code Before Write*/  emitCCAfterWrite=off  CCAfterWrite=/* Custom Code After Write*/  useDMACopy=off  enableBlockingMode=off
  wires:
  Constant13/1 -> data5/1
  Constant5/1 -> data8/1
  Constant3/1 -> data7/1
  Constant2/1 -> data2/1
  Constant1/1 -> data6/1
  Constant/1 -> data1/1
  fault/1 -> Switch1/2, Data Type Conversion3/1
  problem/1 -> Switch1/3, Sum2/2
  Switch1/1 -> data4/1
  Constant4/1 -> Sum2/1
  Sum2/1 -> Switch1/1
  G1or2/1 -> Data Type Conversion8/1
  systate/1 -> Data Type Conversion2/1
  PLL/1 -> Data Type Conversion1/1
  If/1 -> If Action Subsystem/Action
  If Action Subsystem/1(Out1) -> Merge/1
  Merge/1 -> data3/1
  If Action Subsystem1/1(Out1) -> Merge/2
  If Action Subsystem2/1(Out1) -> Merge/3
  If/3 -> If Action Subsystem2/Action
  If/4 -> If Action Subsystem3/Action
  If Action Subsystem3/1(Out1) -> Merge/4
  If/5 -> If Action Subsystem4/Action
  If Action Subsystem4/1(Out1) -> Merge/5
  If Action Subsystem5/1(Out1) -> Merge/6
  If/6 -> If Action Subsystem5/Action
  Data Type Conversion8/1 -> If/2
  Data Type Conversion1/1 -> If/3
  Data Type Conversion2/1 -> If/1
  If Action Subsystem6/1(Out1) -> Merge/7
  If/7 -> If Action Subsystem6/Action
  Data Type Conversion3/1 -> If/4
  If Action Subsystem7/1(Out1) -> Merge/8
  If/8 -> If Action Subsystem7/Action
  If Action Subsystem8/1(Out1) -> Merge/9
  If Action Subsystem9/1(Out1) -> Merge/10
  If Action Subsystem10/1(Out1) -> Merge/11
  If Action Subsystem11/1(Out1) -> Merge/12
  If Action Subsystem12/1(Out1) -> Merge/13
  If Action Subsystem13/1(Out1) -> Merge/14
  If/9 -> If Action Subsystem8/Action
  If/10 -> If Action Subsystem9/Action
  If/11 -> If Action Subsystem10/Action
  If/12 -> If Action Subsystem11/Action
  If/13 -> If Action Subsystem12/Action
  If/2 -> If Action Subsystem1/Action
  If/14 -> If Action Subsystem13/Action
  If/15 -> If Action Subsystem14/Action
  If/16 -> If Action Subsystem15/Action
  If Action Subsystem14/1(Out1) -> Merge/15
  If Action Subsystem15/1(Out1) -> Merge/16

== system Final_V620140905h5b_fuben1/Subsystem5 ==
  In : Inport
  Over_Nr : Inport  Port=2
  B2D : commutil2/Bit to Integer Converter  nbits=8  bitOrder=MSB first  signedOutputValues=Unsigned  outDtype=uint8  outDtypeSigned=Inherit via internal rule
  Constant4 : Constant  Priority=1  Value=[1 1 1 1 1 1 1 0]  OutDataTypeStr=int8
  Constant6 : Constant  Priority=1  Value=[1 1 1 1 1 1 1 1]  OutDataTypeStr=int8
  Logical Operator3 : Logic  AllPortsSameDT=off  OutDataTypeStr=boolean
  Memory Copy : idelinklib_common/Memory Copy  Priority=3  copyFrom=Input port  copyFromAddressSource=Specify via dialog  copyFromAddress=hex2dec('00001000')  copyFromSrcCode=myVariableSrc  dataTypeFrom=uint8  dataDimensionFrom=1  useOffsetFrom=off  offsetFromSrc=Specify via dialog  offsetFrom=0  strideFrom=1  copyTo=Specified address  copyToAddressSource=Specify via dialog  copyToAddress=hex2dec('200010')  copyToSrcCode=myVariableDst  dataTypeTo=int8  useOffsetTo=off  offsetToSrc=Specify via dialog  offsetTo=0  strideTo=1  sampleTime=inf  useInitValue=on  initValueSrc=Specify constant value  initValue=bin2dec('00000000')  initValueSrcCode=myInitValueVariable  useAsMask=off  maskOperator=bitwise AND  useTermValue=on  termValue=bin2dec('00000000')  isRealtimeEnabled=off  emitCCBeforeWrite=off  CCBeforeWrite=/* Custom Code Before Write*/  emitCCAfterWrite=off  CCAfterWrite=/* Custom Code After Write*/  useDMACopy=off  enableBlockingMode=off
  Switch5 : Switch  Criteria=u2 > Threshold  SaturateOnIntegerOverflow=on  InputSameDT=on
  wires:
  B2D/1 -> Memory Copy/1
  Constant4/1 -> Switch5/1
  Constant6/1 -> Switch5/3
  Over_Nr/1 -> Switch5/2
  Switch5/1 -> Logical Operator3/2
  Logical Operator3/1 -> B2D/1
  In/1 -> Logical Operator3/1

== system Final_V620140905h5b_fuben1/Valuble ==
  Ad : idelinklib_common/Memory Allocate  variableName=adtemp1  alignThisVariable=off  memoryAlignmentBoundary=4  dataType=int16  specifyQualifier=off  typeQualifier=volatile  dataDimension=12  specifyMemorySection=off  memorySection=mySEC1  bindMemorySection=on  sectionStartAddress=hex2dec('8000')  initializeMemory=off  initialValue=0
  Ad1 : idelinklib_common/Memory Allocate  variableName=dq  alignThisVariable=off  memoryAlignmentBoundary=4  dataType=int16  specifyQualifier=off  typeQualifier=volatile  dataDimension=1  specifyMemorySection=off  memorySection=mySEC1  bindMemorySection=on  sectionStartAddress=hex2dec('8000')  initializeMemory=off  initialValue=0
  M1 : idelinklib_common/Memory Allocate  variableName=M1  alignThisVariable=off  memoryAlignmentBoundary=4  dataType=int16  specifyQualifier=off  typeQualifier=volatile  dataDimension=1  specifyMemorySection=off  memorySection=mySEC1  bindMemorySection=on  sectionStartAddress=hex2dec('8000')  initializeMemory=off  initialValue=0
  M10 : idelinklib_common/Memory Allocate  variableName=M10  alignThisVariable=off  memoryAlignmentBoundary=4  dataType=int16  specifyQualifier=off  typeQualifier=volatile  dataDimension=1  specifyMemorySection=off  memorySection=mySEC1  bindMemorySection=on  sectionStartAddress=hex2dec('8000')  initializeMemory=off  initialValue=0
  M11 : idelinklib_common/Memory Allocate  variableName=M11  alignThisVariable=off  memoryAlignmentBoundary=4  dataType=int16  specifyQualifier=off  typeQualifier=volatile  dataDimension=1  specifyMemorySection=off  memorySection=mySEC1  bindMemorySection=on  sectionStartAddress=hex2dec('8000')  initializeMemory=off  initialValue=0
  M12 : idelinklib_common/Memory Allocate  variableName=M12  alignThisVariable=off  memoryAlignmentBoundary=4  dataType=int16  specifyQualifier=off  typeQualifier=volatile  dataDimension=1  specifyMemorySection=off  memorySection=mySEC1  bindMemorySection=on  sectionStartAddress=hex2dec('8000')  initializeMemory=off  initialValue=0
  M2 : idelinklib_common/Memory Allocate  variableName=M2  alignThisVariable=off  memoryAlignmentBoundary=4  dataType=int16  specifyQualifier=off  typeQualifier=volatile  dataDimension=1  specifyMemorySection=off  memorySection=mySEC1  bindMemorySection=on  sectionStartAddress=hex2dec('8000')  initializeMemory=off  initialValue=0
  M3 : idelinklib_common/Memory Allocate  variableName=M3  alignThisVariable=off  memoryAlignmentBoundary=4  dataType=int16  specifyQualifier=off  typeQualifier=volatile  dataDimension=1  specifyMemorySection=off  memorySection=mySEC1  bindMemorySection=on  sectionStartAddress=hex2dec('8000')  initializeMemory=off  initialValue=0
  M4 : idelinklib_common/Memory Allocate  variableName=M4  alignThisVariable=off  memoryAlignmentBoundary=4  dataType=int16  specifyQualifier=off  typeQualifier=volatile  dataDimension=1  specifyMemorySection=off  memorySection=mySEC1  bindMemorySection=on  sectionStartAddress=hex2dec('8000')  initializeMemory=off  initialValue=0
  M5 : idelinklib_common/Memory Allocate  variableName=M5  alignThisVariable=off  memoryAlignmentBoundary=4  dataType=int16  specifyQualifier=off  typeQualifier=volatile  dataDimension=1  specifyMemorySection=off  memorySection=mySEC1  bindMemorySection=on  sectionStartAddress=hex2dec('8000')  initializeMemory=off  initialValue=0
  M6 : idelinklib_common/Memory Allocate  variableName=M6  alignThisVariable=off  memoryAlignmentBoundary=4  dataType=int16  specifyQualifier=off  typeQualifier=volatile  dataDimension=1  specifyMemorySection=off  memorySection=mySEC1  bindMemorySection=on  sectionStartAddress=hex2dec('8000')  initializeMemory=off  initialValue=0
  M7 : idelinklib_common/Memory Allocate  variableName=M7  alignThisVariable=off  memoryAlignmentBoundary=4  dataType=int16  specifyQualifier=off  typeQualifier=volatile  dataDimension=1  specifyMemorySection=off  memorySection=mySEC1  bindMemorySection=on  sectionStartAddress=hex2dec('8000')  initializeMemory=off  initialValue=0
  M8 : idelinklib_common/Memory Allocate  variableName=M8  alignThisVariable=off  memoryAlignmentBoundary=4  dataType=int16  specifyQualifier=off  typeQualifier=volatile  dataDimension=1  specifyMemorySection=off  memorySection=mySEC1  bindMemorySection=on  sectionStartAddress=hex2dec('8000')  initializeMemory=off  initialValue=0
  M9 : idelinklib_common/Memory Allocate  variableName=M9  alignThisVariable=off  memoryAlignmentBoundary=4  dataType=int16  specifyQualifier=off  typeQualifier=volatile  dataDimension=1  specifyMemorySection=off  memorySection=mySEC1  bindMemorySection=on  sectionStartAddress=hex2dec('8000')  initializeMemory=off  initialValue=0
  wave2 : idelinklib_common/Memory Allocate  variableName=wave2  alignThisVariable=off  memoryAlignmentBoundary=4  dataType=int16  specifyQualifier=off  typeQualifier=volatile  dataDimension=1000  specifyMemorySection=off  memorySection=mySEC1  bindMemorySection=on  sectionStartAddress=hex2dec('8000')  initializeMemory=off  initialValue=0
  wave3 : idelinklib_common/Memory Allocate  variableName=wave3  alignThisVariable=off  memoryAlignmentBoundary=4  dataType=int16  specifyQualifier=off  typeQualifier=volatile  dataDimension=1000  specifyMemorySection=off  memorySection=mySEC1  bindMemorySection=on  sectionStartAddress=hex2dec('8000')  initializeMemory=off  initialValue=0

== system Final_V620140905h5b_fuben1/action for state0 ==
  note: The fourth one is for load switch 0 is on
  note: The last one is for protect 0 is protect
  note: The sixth one is for Q2 on singal, 0 is on when the Q2 wants to be turned off, the i/o must be set to 1
  note: The third one is for Q2 off singal, 0 is off when the Q2 wants to be turned on, the i/o must be set to 1
  note: 0 is Q2 and Q3 off;2 is Q2 on;1 is Q3 on;3 is Q2 on
  Action Port : ActionPort  ActionType=case
  Constant1 : Constant  Priority=1  Value=0  OutDataTypeStr=boolean
  Constant2 : Constant  Priority=1  Value=[1 1 1 1 1 1 1 1]  OutDataTypeStr=int8
  Digital Output : c2833xlib/Digital Output  Tag=1  Priority=2  GPIO_Number=GPIO8~GPIO15  GPIO_Bit0=off  GPIO_BIT0_Toggle=off  GPIO_Bit1=off  GPIO_BIT1_Toggle=off  GPIO_Bit2=off  GPIO_BIT2_Toggle=off  GPIO_Bit3=off  GPIO_BIT3_Toggle=off  GPIO_Bit4=on  GPIO_BIT4_Toggle=off  GPIO_Bit5=off  GPIO_BIT5_Toggle=off  GPIO_Bit6=off  GPIO_BIT6_Toggle=off  GPIO_Bit7=off  GPIO_BIT7_Toggle=off
  Out : Outport
  wires:
  Constant1/1 -> Digital Output/1
  Constant2/1 -> Out/1
